simulink model "testEIS"  (R2022a)
settings: Solver=VariableStepAuto  StartTime=0.0  StopTime=Inf  MaxStep=1e-4  RelTol=1e-3
undefined symbols (not defined in the file): Call, Function, Neg, Pos
libraries: fl_lib x1, nesl_utility x1
settings Model: Creator=mmarq  LastModifiedBy=mmarq
settings SolverCC: ZeroCrossAlgorithm=Adaptive
settings DebuggingCC: IgnoredZcDiagnostic=none

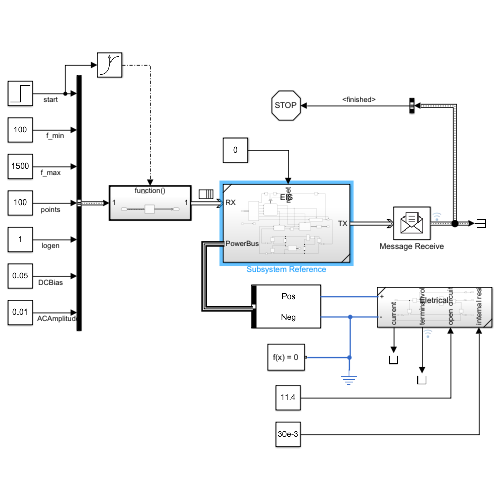
[thumbnail: Simulink's stored preview of the top-level diagram]
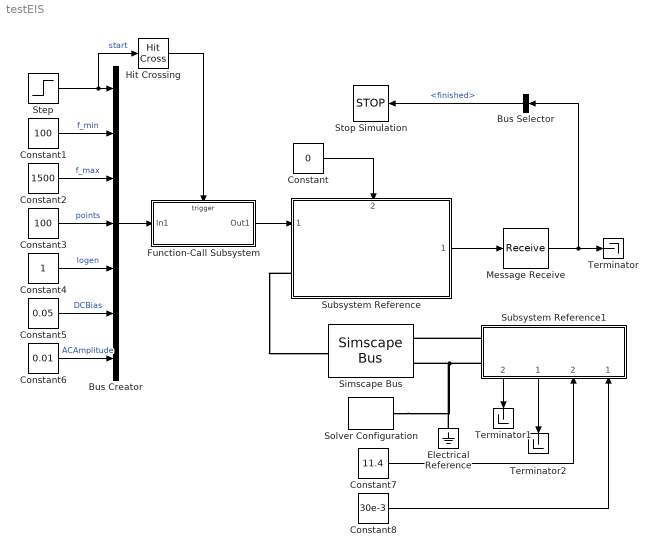
== system testEIS ==
  Bus Creator : BusCreator  Inputs=7  OutDataTypeStr=Bus: EISCmd  NonVirtualBus=on
      settings: InheritFromInputs=off
  Bus Selector : BusSelector  OutputSignals=finished
  Constant : Constant  Value=0
  Constant1 : Constant  Value=100
  Constant2 : Constant  Value=1500
  Constant3 : Constant  Value=100
  Constant4 : Constant
  Constant5 : Constant  Value=0.05
  Constant6 : Constant  Value=0.01
  Constant7 : Constant  Value=11.4
  Constant8 : Constant  Value=30e-3
  Electrical Reference : fl_lib/Electrical/Electrical Elements/Electrical Reference
      settings: SourceProductBaseCode=PW,SS,VE
  Function-Call Subsystem : Subsystem  TreatAsAtomicUnit=on
  Hit Crossing : HitCross  HitCrossingOffset=0.01  HitCrossingDirection=rising  HitCrossingOutputType=Function-Call
  Message Receive : Receive  InputPortMessageModes=m  ValueSourceWhenQueueIsEmpty=Use initial value
  Simscape Bus : SimscapeBus  HierarchyStrings=Pos;Neg
  Solver Configuration : nesl_utility/Solver Configuration  PhysicalDomain=network_engine_domain  SubClassName=solver  LeftPortType=input  RightPortType=generic  Tones=[]  Harmonics=[]  SimulateNoise=off  Profile=off  UseLocalSampling=off  EnableSwitchedLinearOptims=on  FrequencyDomain=off  UseCCode=off  RelTol=0.001  AbsTol=0.001  MinStep=1e-09  ToWorkspace=off  RevertToSquareIcSolve=off  NumHomotopyIterations=100  PhasorMode=off  PhasorModeNumHarmonics=1  IndexReductionMethod=DerivativeReplacement  DoDC=on  ResidualTolerance=1e-09  UseLocalSolver=off  LocalSolverChoice=NE_BACKWARD_EULER_ADVANCER  LocalSolverSampleTime=0.001  DoFixedCost=off  MaxNonlinIter=3  MaxModeIter=2  ComputeImpulses=off  ImpulseIterations=2  LinearAlgebra=auto  LinearAlgebraNumThread=0  EquationFormulation=NE_TIME_EF  DelaysMemoryBudget=1024  AutomaticFiltering=on  FilteringTimeConstant=0.001  PartitionStorageMethod=AS_NEEDED  PartitionMemoryBudget=1024  PartitionMethod=ROBUST
      settings: SourceProductBaseCode=SS,PW,VE
  Step : Step  SampleTime=0
  Stop Simulation : Stop
  Subsystem Reference : Subsystem  ReferencedSubsystem=EIS
      settings: PortSchema="{\"entries\":[{\"content\":{\"sides\":[{\"content\":{\"connectorIds\":[\"In1\",\"LConn1\"]},\"type\":\"ConnectorPlacement.EquallySpacedRectSide\",\"uuid\":\"bda901de-5fc5-4df6-bed4-bf969933d972\"},{\"content\":{\"connectorIds\":[\"Out1\"],\"side\":\"RIGHT\"},\"type\":\"ConnectorPlacement.EquallySpacedRectSide\",\"uuid\":\"97e6e5df-6a68-4cb9-aa40-ad9555eae5d3\"},{\"content\":{\"connectorIds\":[\"In2\"],\"side\":\"TOP\"},\"type\":\"ConnectorPlacement.EquallySpacedRectSide\",\"uuid\":\"3686a2fc-9119-406b-ac45-90d58aa6d823\"}]},\"type\":\"ConnectorPlacement.EquallySpacedConnector\",\"uuid\":\"6daecac9-5e0e-4dc6-b323-39bbe07465b3\"}],\"packageUris\":[\"http://schema.mathworks.com/mf0/Connector/R2020b\"],\"version\":\"1.0\"}"
  Subsystem Reference1 : Subsystem  ReferencedSubsystem=Eletrical
      settings: PortSchema="{\"entries\":[{\"content\":{\"sides\":[{\"content\":{\"connectorIds\":[\"LConn1\",\"LConn2\"]},\"type\":\"ConnectorPlacement.EquallySpacedRectSide\",\"uuid\":\"18f53ad7-56e7-49d9-b972-037d4274abd2\"},{\"content\":{\"connectorIds\":[],\"side\":\"RIGHT\"},\"type\":\"ConnectorPlacement.EquallySpacedRectSide\",\"uuid\":\"c8641c6f-84a2-459f-b0c5-5f970ee05955\"},{\"content\":{\"connectorIds\":[],\"side\":\"TOP\"},\"type\":\"ConnectorPlacement.EquallySpacedRectSide\",\"uuid\":\"f7d0a8d0-9d27-478a-a0c8-3d46e120ece0\"},{\"content\":{\"connectorIds\":[\"Out2\",\"Out1\",\"In2\",\"In1\"],\"side\":\"BOTTOM\"},\"type\":\"ConnectorPlacement.EquallySpacedRectSide\",\"uuid\":\"2a24cac0-8444-43f8-bdfe-3a905fb450b1\"}]},\"type\":\"ConnectorPlacement.EquallySpacedConnector\",\"uuid\":\"1e93c122-0500-4305-b316-cc64e5086090\"}],\"packageUris\":[\"http://schema.mathworks.com/mf0/Connector/R2020b\"],\"version\":\"1.0\"}"
  Terminator : Terminator
  Terminator1 : Terminator
  Terminator2 : Terminator
  wires:
  Step/1 -> Hit Crossing/1, Bus Creator/1  "start"
  Constant1/1 -> Bus Creator/2  "f_min"
  Constant2/1 -> Bus Creator/3  "f_max"
  Constant3/1 -> Bus Creator/4  "points"
  Constant4/1 -> Bus Creator/5  "logen"
  Constant5/1 -> Bus Creator/6  "DCBias"
  Constant6/1 -> Bus Creator/7  "ACAmplitude"
  Subsystem Reference/1 -> Message Receive/1
  Bus Creator/1 -> Function-Call Subsystem/1(In1)
  Function-Call Subsystem/1(Out1) -> Subsystem Reference/1
  Hit Crossing/1 -> Function-Call Subsystem/Trigger
  Message Receive/1 -> Bus Selector/1, Terminator/1
  Bus Selector/1 -> Stop Simulation/1  "<finished>"
  Constant/1 -> Subsystem Reference/2
  Subsystem Reference1/2 -> Terminator1/1
  Subsystem Reference1/1 -> Terminator2/1
  Constant7/1 -> Subsystem Reference1/2
  Constant8/1 -> Subsystem Reference1/1
  connections:
  Subsystem Reference/LConn1 -- Simscape Bus/RConn1
  Subsystem Reference1/LConn1 -- Simscape Bus/LConn1
  Subsystem Reference1/LConn2 -- Electrical Reference/LConn1 -- Solver Configuration/RConn1 -- Simscape Bus/LConn2

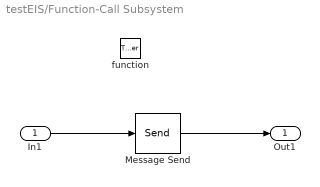
== system testEIS/Function-Call Subsystem ==
  In1 : Inport
  function : TriggerPort  TriggerType=function-call  VariantControl=(inherit)
  Message Send : Send  OutputPortMessageModes=m
  Out1 : Outport
  wires:
  In1/1 -> Message Send/1
  Message Send/1 -> Out1/1
